simulink model "complexfft4"  (R2021b)
settings: Solver=VariableStepAuto  StartTime=0.0  StopTime=10.0  RelTol=1e-3
libraries: hdlBasic x34, xbsIndex_r4 x1
settings Model: Creator=Apoorv  LastModifiedBy=Apoorv

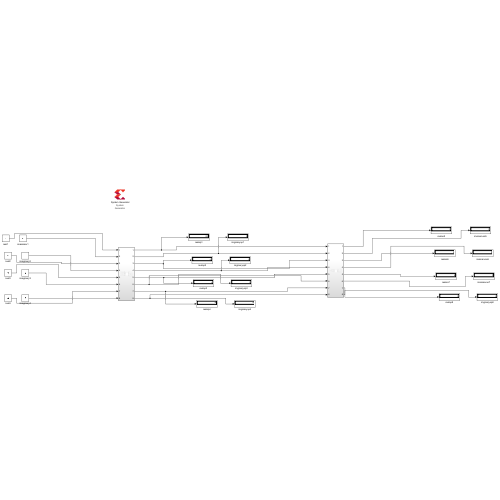
[thumbnail: Simulink's stored preview of the top-level diagram]
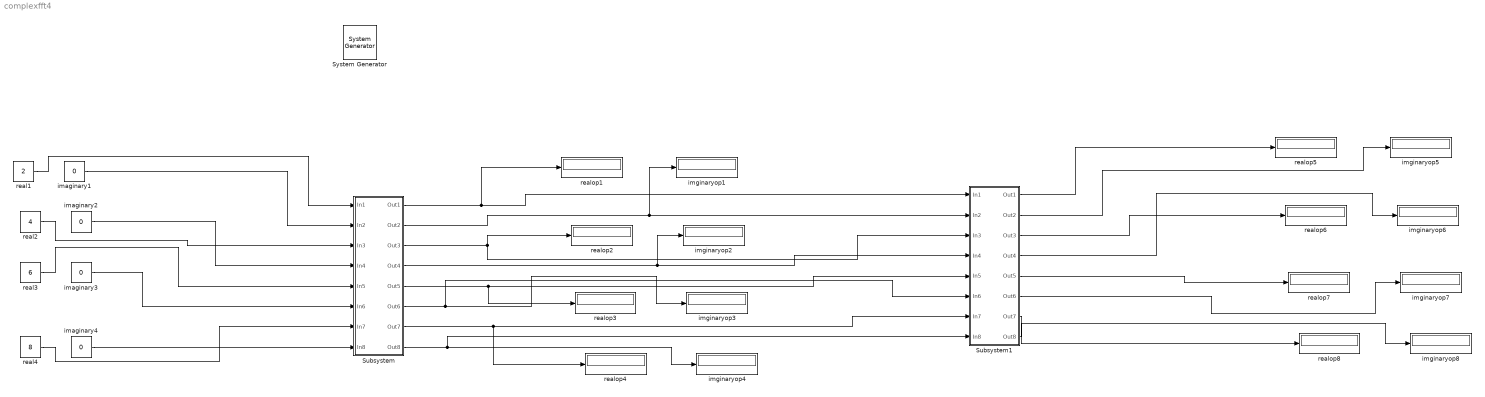
== system complexfft4 ==
  " System Generator" : xbsIndex_r4/ System Generator  Tag=genX  xilinxfamily=kintex7  part=xc7k160t  speed=-1  package=fbg484  synthesis_tool=Vivado  clock_wrapper=Clock Enables  directory=./netlist  proj_type=Vivado  Synth_file=Vivado Synthesis Defaults  Impl_file=Vivado Implementation Defaults  testbench=off  simulink_period=1  sysclk_period=10  dcm_input_clock_period=10  incr_netlist=off  trim_vbits=Everywhere in SubSystem  dbl_ovrd=According to Block Masks  core_generation=According to Block Masks  run_coregen=off  deprecated_control=off  eval_field=0  block_type=sysgen
  Subsystem : Subsystem
  Subsystem1 : Subsystem
  imaginary{1..4} (4 alike) : Constant  Value=0
  imginaryop{1..8} (8 alike) : Display
      settings: Format=decimal (Stored Integer)
  real1 : Constant  Value=2
  real2 : Constant  Value=4
  real3 : Constant  Value=6
  real4 : Constant  Value=8
  realop{1..8} (8 alike) : Display
      settings: Format=decimal (Stored Integer)
  wires:
  Subsystem/6(Out6) -> Subsystem1/6(In6), imginaryop3/1
  Subsystem/8(Out8) -> imginaryop4/1, Subsystem1/8(In8)
  Subsystem/7(Out7) -> Subsystem1/7(In7), realop4/1
  Subsystem/4(Out4) -> Subsystem1/4(In4), imginaryop2/1
  Subsystem/5(Out5) -> Subsystem1/5(In5), realop3/1
  Subsystem/1(Out1) -> Subsystem1/1(In1), realop1/1
  Subsystem/3(Out3) -> Subsystem1/3(In3), realop2/1
  Subsystem/2(Out2) -> Subsystem1/2(In2), imginaryop1/1
  real1/1 -> Subsystem/1(In1)
  imaginary1/1 -> Subsystem/2(In2)
  real2/1 -> Subsystem/3(In3)
  imaginary2/1 -> Subsystem/4(In4)
  real3/1 -> Subsystem/5(In5)
  imaginary3/1 -> Subsystem/6(In6)
  real4/1 -> Subsystem/7(In7)
  imaginary4/1 -> Subsystem/8(In8)
  Subsystem1/1(Out1) -> realop5/1
  Subsystem1/2(Out2) -> imginaryop5/1
  Subsystem1/3(Out3) -> realop6/1
  Subsystem1/4(Out4) -> imginaryop6/1
  Subsystem1/5(Out5) -> realop7/1
  Subsystem1/6(Out6) -> imginaryop7/1
  Subsystem1/7(Out7) -> realop8/1
  Subsystem1/8(Out8) -> imginaryop8/1

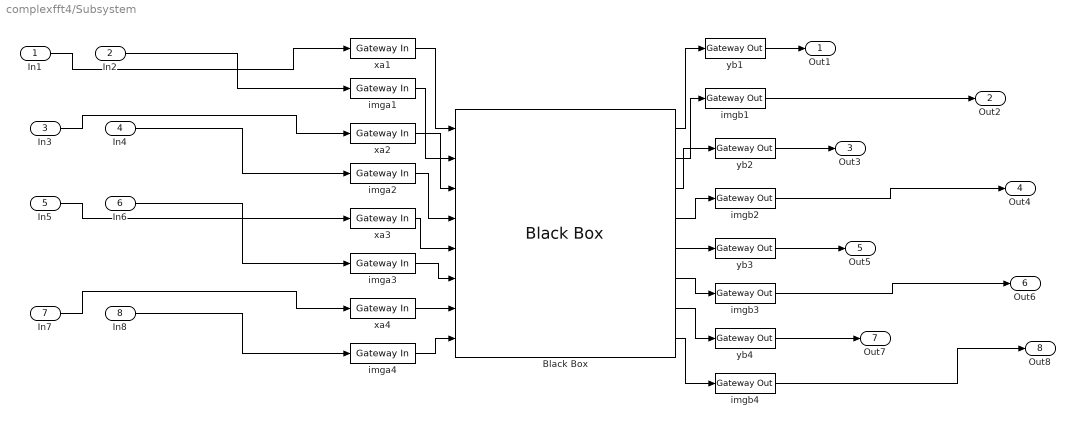
== system complexfft4/Subsystem ==
  In1 : Inport
  In2 : Inport  Port=2
  In3 : Inport  Port=3
  In4 : Inport  Port=4
  In5 : Inport  Port=5
  In6 : Inport  Port=6
  In7 : Inport  Port=7
  In8 : Inport  Port=8
  Black Box : hdlBasic/Black Box  init_code=compff4_config  sim_method=Vivado Simulator  verbose=off  XmcBlockStatus=1  maskContainerNames=group1  block_type=blackbox2  block_config=sysgen:black_box_config
  imga{1..4} (4 alike) : hdlBasic/Gateway In  gui_display_data_type=Fixed-point  arith_type=Signed (2's comp)  n_bits=8  bin_pt=0  preci_type=Single  exp_width=8  frac_width=24  rows=1  columns=1  quantization="Round  (unbiased: +/- Inf)"  overflow=Saturate  period=1  UseAsADC=off  ADCChannel='1'  interface=None  automatic_assignment=on  address_offset=hex2dec('00')  intf_name=''  intf_description=''  default_value=0  timing_constraint=None  locs_specified=off  LOCs={}  io_standard={}  inherit_from_input=off  hdl_port=on  XmcBlockStatus=1  maskContainerNames=group4  block_type=gatewayin  block_config=sysgen:gateway_in_config  block_width_w=590  block_height_w=620  block_width=640  block_height=850
  imgb{1..4} (4 alike) : hdlBasic/Gateway Out  inherit_from_input=on  hdl_port=off  rows=1  columns=1  UseAsDAC=off  DACChannel='1'  interface=None  automatic_assignment=on  address_offset=hex2dec('00')  intf_name=''  intf_description=''  timing_constraint=None  locs_specified=off  LOCs={}  io_standard={}  XmcBlockStatus=1  maskContainerNames=group4  block_type=gatewayout  block_config=sysgen:gateway_out_config  block_width_w=590  block_height_w=620  block_width=620  block_height=750
  xa{1..4} (4 alike) : hdlBasic/Gateway In  gui_display_data_type=Fixed-point  arith_type=Signed (2's comp)  n_bits=8  bin_pt=0  preci_type=Single  exp_width=8  frac_width=24  rows=1  columns=1  quantization="Round  (unbiased: +/- Inf)"  overflow=Saturate  period=1  UseAsADC=off  ADCChannel='1'  interface=None  automatic_assignment=on  address_offset=hex2dec('00')  intf_name=''  intf_description=''  default_value=0  timing_constraint=None  locs_specified=off  LOCs={}  io_standard={}  inherit_from_input=off  hdl_port=on  XmcBlockStatus=1  maskContainerNames=group4  block_type=gatewayin  block_config=sysgen:gateway_in_config  block_width_w=590  block_height_w=620  block_width=640  block_height=850
  yb{1..4} (4 alike) : hdlBasic/Gateway Out  inherit_from_input=on  hdl_port=off  rows=1  columns=1  UseAsDAC=off  DACChannel='1'  interface=None  automatic_assignment=on  address_offset=hex2dec('00')  intf_name=''  intf_description=''  timing_constraint=None  locs_specified=off  LOCs={}  io_standard={}  XmcBlockStatus=1  maskContainerNames=group4  block_type=gatewayout  block_config=sysgen:gateway_out_config  block_width_w=590  block_height_w=620  block_width=620  block_height=750
  Out1 : Outport
  Out2 : Outport  Port=2
  Out3 : Outport  Port=3
  Out4 : Outport  Port=4
  Out5 : Outport  Port=5
  Out6 : Outport  Port=6
  Out7 : Outport  Port=7
  Out8 : Outport  Port=8
  wires:
  Black Box/1 -> yb1/1
  imga1/1 -> Black Box/2
  Black Box/6 -> imgb3/1
  In5/1 -> xa3/1
  xa4/1 -> Black Box/7
  imga4/1 -> Black Box/8
  xa2/1 -> Black Box/3
  imga3/1 -> Black Box/6
  Black Box/5 -> yb3/1
  Black Box/3 -> yb2/1
  Black Box/8 -> imgb4/1
  Black Box/2 -> imgb1/1
  imga2/1 -> Black Box/4
  Black Box/4 -> imgb2/1
  xa1/1 -> Black Box/1
  Black Box/7 -> yb4/1
  yb3/1 -> Out5/1
  xa3/1 -> Black Box/5
  In4/1 -> imga2/1
  In6/1 -> imga3/1
  In7/1 -> xa4/1
  In8/1 -> imga4/1
  yb1/1 -> Out1/1
  In2/1 -> imga1/1
  yb2/1 -> Out3/1
  imgb2/1 -> Out4/1
  imgb1/1 -> Out2/1
  imgb3/1 -> Out6/1
  imgb4/1 -> Out8/1
  yb4/1 -> Out7/1
  In1/1 -> xa1/1
  In3/1 -> xa2/1

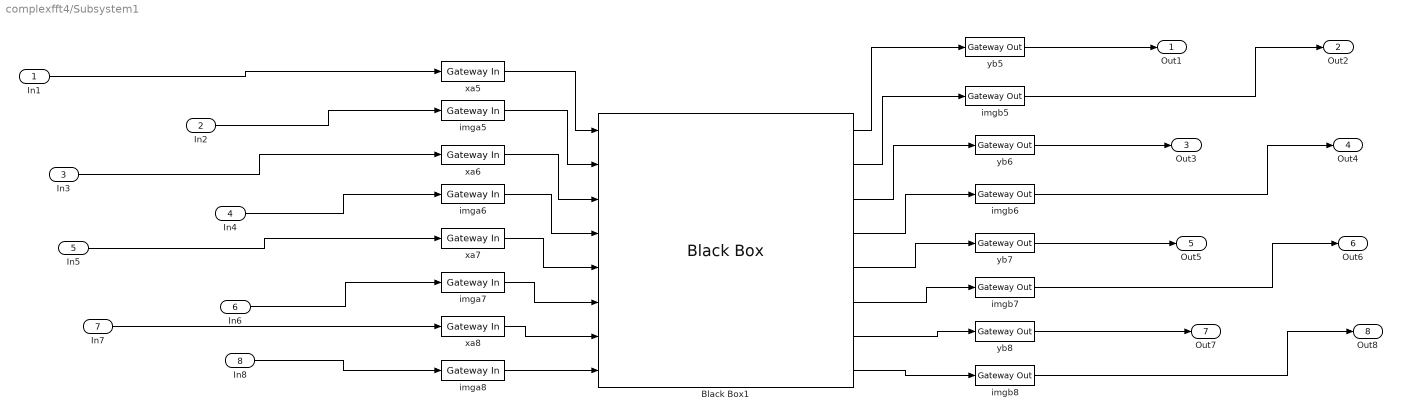
== system complexfft4/Subsystem1 ==
  In1 : Inport
  In2 : Inport  Port=2
  In3 : Inport  Port=3
  In4 : Inport  Port=4
  In5 : Inport  Port=5
  In6 : Inport  Port=6
  In7 : Inport  Port=7
  In8 : Inport  Port=8
  Black Box1 : hdlBasic/Black Box  init_code=compifft4_config  sim_method=Vivado Simulator  verbose=off  XmcBlockStatus=1  maskContainerNames=group1  block_type=blackbox2  block_config=sysgen:black_box_config
  imga{5..8} (4 alike) : hdlBasic/Gateway In  gui_display_data_type=Fixed-point  arith_type=Signed (2's comp)  n_bits=8  bin_pt=0  preci_type=Single  exp_width=8  frac_width=24  rows=1  columns=1  quantization="Round  (unbiased: +/- Inf)"  overflow=Saturate  period=1  UseAsADC=off  ADCChannel='1'  interface=None  automatic_assignment=on  address_offset=hex2dec('00')  intf_name=''  intf_description=''  default_value=0  timing_constraint=None  locs_specified=off  LOCs={}  io_standard={}  inherit_from_input=off  hdl_port=on  XmcBlockStatus=1  maskContainerNames=group4  block_type=gatewayin  block_config=sysgen:gateway_in_config  block_width_w=590  block_height_w=620  block_width=640  block_height=850
  imgb{5..8} (4 alike) : hdlBasic/Gateway Out  inherit_from_input=on  hdl_port=off  rows=1  columns=1  UseAsDAC=off  DACChannel='1'  interface=None  automatic_assignment=on  address_offset=hex2dec('00')  intf_name=''  intf_description=''  timing_constraint=None  locs_specified=off  LOCs={}  io_standard={}  XmcBlockStatus=1  maskContainerNames=group4  block_type=gatewayout  block_config=sysgen:gateway_out_config  block_width_w=590  block_height_w=620  block_width=620  block_height=750
  xa{5..8} (4 alike) : hdlBasic/Gateway In  gui_display_data_type=Fixed-point  arith_type=Signed (2's comp)  n_bits=8  bin_pt=0  preci_type=Single  exp_width=8  frac_width=24  rows=1  columns=1  quantization="Round  (unbiased: +/- Inf)"  overflow=Saturate  period=1  UseAsADC=off  ADCChannel='1'  interface=None  automatic_assignment=on  address_offset=hex2dec('00')  intf_name=''  intf_description=''  default_value=0  timing_constraint=None  locs_specified=off  LOCs={}  io_standard={}  inherit_from_input=off  hdl_port=on  XmcBlockStatus=1  maskContainerNames=group4  block_type=gatewayin  block_config=sysgen:gateway_in_config  block_width_w=590  block_height_w=620  block_width=640  block_height=850
  yb{5..8} (4 alike) : hdlBasic/Gateway Out  inherit_from_input=on  hdl_port=off  rows=1  columns=1  UseAsDAC=off  DACChannel='1'  interface=None  automatic_assignment=on  address_offset=hex2dec('00')  intf_name=''  intf_description=''  timing_constraint=None  locs_specified=off  LOCs={}  io_standard={}  XmcBlockStatus=1  maskContainerNames=group4  block_type=gatewayout  block_config=sysgen:gateway_out_config  block_width_w=590  block_height_w=620  block_width=620  block_height=750
  Out1 : Outport
  Out2 : Outport  Port=2
  Out3 : Outport  Port=3
  Out4 : Outport  Port=4
  Out5 : Outport  Port=5
  Out6 : Outport  Port=6
  Out7 : Outport  Port=7
  Out8 : Outport  Port=8
  wires:
  Black Box1/4 -> imgb6/1
  xa5/1 -> Black Box1/1
  imga6/1 -> Black Box1/4
  imga5/1 -> Black Box1/2
  Black Box1/2 -> imgb5/1
  xa6/1 -> Black Box1/3
  Black Box1/1 -> yb5/1
  yb7/1 -> Out5/1
  In3/1 -> xa6/1
  Black Box1/8 -> imgb8/1
  xa7/1 -> Black Box1/5
  Black Box1/3 -> yb6/1
  imga7/1 -> Black Box1/6
  imga8/1 -> Black Box1/8
  xa8/1 -> Black Box1/7
  imgb5/1 -> Out2/1
  In7/1 -> xa8/1
  Black Box1/6 -> imgb7/1
  Black Box1/7 -> yb8/1
  Black Box1/5 -> yb7/1
  In8/1 -> imga8/1
  In1/1 -> xa5/1
  In4/1 -> imga6/1
  In5/1 -> xa7/1
  In6/1 -> imga7/1
  In2/1 -> imga5/1
  imgb7/1 -> Out6/1
  yb6/1 -> Out3/1
  imgb6/1 -> Out4/1
  imgb8/1 -> Out8/1
  yb5/1 -> Out1/1
  yb8/1 -> Out7/1
